simulink model "rules2"  (R2016a)
settings: Solver=VariableStepAuto  StartTime=0.0  StopTime=50  RelTol=1e-3
libraries: simulink x5, fuzblock x5
settings Model: Creator=SPDKH  LastModifiedBy=SPDKH

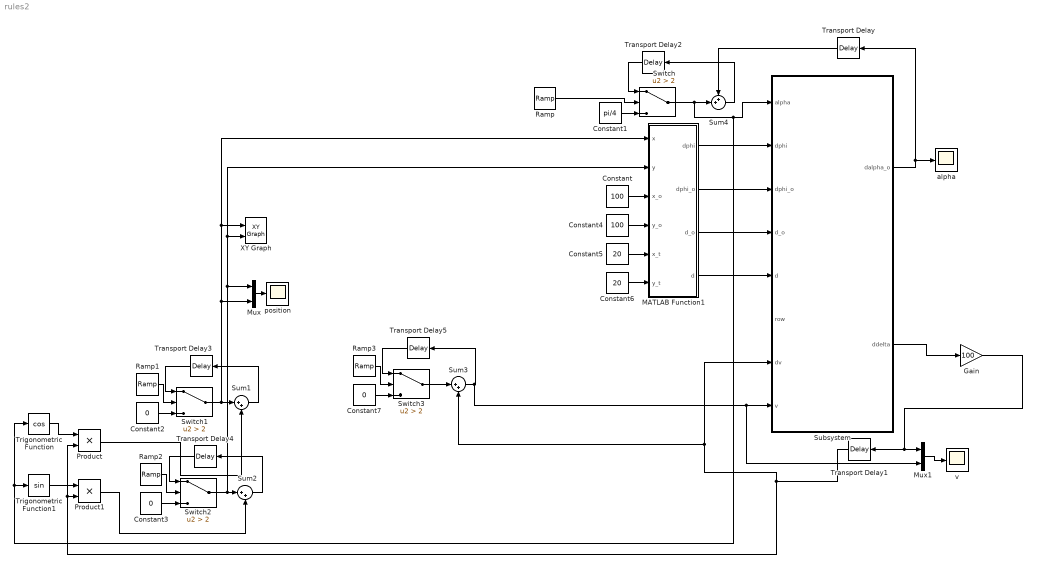
== system rules2 ==
  Constant : Constant  Value=100
  Constant1 : Constant  Value=pi/4
  Constant2 : Constant  Value=0
  Constant3 : Constant  Value=0
  Constant4 : Constant  Value=100
  Constant5 : Constant  Value=20
  Constant6 : Constant  Value=20
  Constant7 : Constant  Value=0
  Gain : Gain  Gain=100
  MATLAB Function1 : MATLAB Function  TreatAsAtomicUnit=on
  Mux : Mux  Inputs=2
  Mux1 : Mux  Inputs=2
  Product : Product
  Product1 : Product
  Ramp{,1..3} (4 alike) : simulink/Sources/Ramp  slope=1  start=0  X0=0
  Subsystem : Subsystem
  Sum1 : Sum  Inputs=|++
  Sum2 : Sum  Inputs=|++
  Sum3 : Sum  Inputs=|++
  Sum4 : Sum  Inputs=++|
  Switch{,1..3} (4 alike) : Switch  Criteria=u2 > Threshold  Threshold=2
  Transport Delay : TransportDelay  DelayTime=0.001  TransDelayFeedthrough=on
  Transport Delay{1,3..5} (4 alike) : TransportDelay
  Transport Delay2 : TransportDelay  TransDelayFeedthrough=on
  Trigonometric Function : Trigonometry  Operator=cos
  Trigonometric Function1 : Trigonometry
  XY Graph : simulink/Sinks/XY Graph  xmin=-10  xmax=100  ymin=-10  ymax=100  st=-1
  alpha : Scope
  position : Scope
  v : Scope
  wires:
  Subsystem/1("dalpha_o ") -> alpha/1, Transport Delay/1
  MATLAB Function1/4(d) -> Subsystem/5(d)
  MATLAB Function1/3(d_o) -> Subsystem/4(d_o)
  MATLAB Function1/2(dphi_o) -> Subsystem/3("dphi_o ")
  MATLAB Function1/1(dphi) -> Subsystem/2("dphi ")
  Constant1/1 -> Switch/3
  Ramp/1 -> Switch/2
  Constant2/1 -> Switch1/3
  Transport Delay3/1 -> Switch1/1
  Ramp1/1 -> Switch1/2
  Switch1/1 -> Mux/2, XY Graph/1, MATLAB Function1/1(x), Sum1/1
  Sum1/1 -> Transport Delay3/1
  Constant3/1 -> Switch2/3
  Transport Delay4/1 -> Switch2/1
  Ramp2/1 -> Switch2/2
  Sum2/1 -> Transport Delay4/1
  Constant/1 -> MATLAB Function1/3(x_o)
  Constant4/1 -> MATLAB Function1/4(y_o)
  Constant5/1 -> MATLAB Function1/5(x_t)
  Constant6/1 -> MATLAB Function1/6(y_t)
  Mux/1 -> position/1
  Constant7/1 -> Switch3/3
  Transport Delay5/1 -> Switch3/1
  Ramp3/1 -> Switch3/2
  Sum3/1 -> Mux1/2, Subsystem/8(v), Transport Delay5/1
  Switch3/1 -> Sum3/1
  Mux1/1 -> v/1
  Transport Delay/1 -> Sum4/1
  Transport Delay2/1 -> Switch/1
  Sum4/1 -> Transport Delay2/1
  Switch2/1 -> Mux/1, XY Graph/2, MATLAB Function1/2(y), Sum2/1
  Subsystem/2(ddelta) -> Gain/1
  Gain/1 -> Transport Delay1/1, Mux1/1
  Trigonometric Function/1 -> Product/1
  Trigonometric Function1/1 -> Product1/1
  Switch/1 -> Trigonometric Function/1, Trigonometric Function1/1, Subsystem/1(alpha), Sum4/2
  Product/1 -> Sum1/2
  Product1/1 -> Sum2/2
  Transport Delay1/1 -> Product1/2, Product/2, Sum3/2, Subsystem/7(dv)

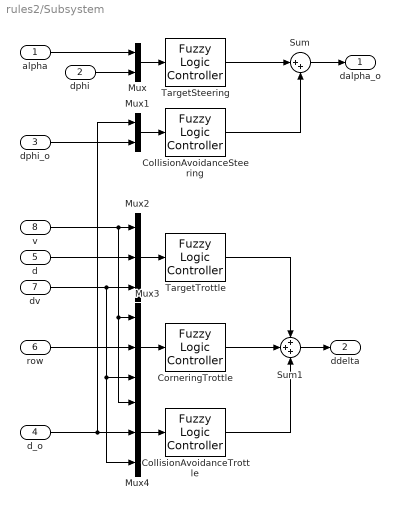
== system rules2/Subsystem ==
  alpha : Inport
  "dphi " : Inport  Port=2
  "dphi_o " : Inport  Port=3
  d_o : Inport  Port=4
  d : Inport  Port=5
  row : Inport  Port=6
  dv : Inport  Port=7
  v : Inport  Port=8
  "CollisionAvoidanceSteering " : fuzblock/Fuzzy Logic  Controller  fis=['CollisionAvoidanceSteering.fis']
  "CollisionAvoidanceTrottle " : fuzblock/Fuzzy Logic  Controller  fis=['CollisionAvoidanceThrottle.fis']
  "CorneringTrottle " : fuzblock/Fuzzy Logic  Controller  fis=['CorneringTrottle.fis']
  Mux : Mux  Inputs=2
  Mux1 : Mux  Inputs=2
  Mux2 : Mux  Inputs=3
  Mux3 : Mux  Inputs=3
  Mux4 : Mux  Inputs=3
  Sum : Sum  Inputs=|++
  Sum1 : Sum  Inputs=+++
  TargetSteering : fuzblock/Fuzzy Logic  Controller  fis=['TargetSteering2.fis']
  TargetTrottle : fuzblock/Fuzzy Logic  Controller  fis=['TargetTrottle.fis']
  "dalpha_o " : Outport
  ddelta : Outport  Port=2
  wires:
  TargetTrottle/1 -> Sum1/1
  "CorneringTrottle "/1 -> Sum1/2
  "CollisionAvoidanceTrottle "/1 -> Sum1/3
  TargetSteering/1 -> Sum/1
  "CollisionAvoidanceSteering "/1 -> Sum/2
  Mux/1 -> TargetSteering/1
  Mux1/1 -> "CollisionAvoidanceSteering "/1
  Mux2/1 -> TargetTrottle/1
  Mux3/1 -> "CorneringTrottle "/1
  Mux4/1 -> "CollisionAvoidanceTrottle "/1
  v/1 -> Mux4/1, Mux3/1, Mux2/1
  d/1 -> Mux2/2
  dv/1 -> Mux4/3, Mux3/3, Mux2/3
  row/1 -> Mux3/2
  d_o/1 -> Mux1/1, Mux4/2
  alpha/1 -> Mux/1
  "dphi "/1 -> Mux/2
  "dphi_o "/1 -> Mux1/2
  Sum/1 -> "dalpha_o "/1
  Sum1/1 -> ddelta/1

== matlab function rules2/MATLAB Function1 ==
  data: dphi output; dphi_o output; d_o output; x input; d output; y input; x_o input; y_o input; x_t input; y_t input
function [dphi,dphi_o,d_o,d] = fcn(x,y,x_o,y_o,x_t,y_t)

 if ((x_t-x) < 0)
     dphi = atan ((y_t-y)/(x_t-x))+pi;
 else 
    dphi = atan ((y_t-y)/(x_t-x));
 end
 
 if ((x_o-x) < 0)
     dphi_o = atan ((y_o-y)/(x_o-x));+pi;
 else 
    dphi_o = atan ((y_o-y)/(x_o-x));
 end


d_o = norm([(x_o-x),(y_o-y)]);
d = norm([(x_t-x),(y_t-y)]);
